simulink library "thc"  (R2021b)
settings: Solver=VariableStepAuto  StartTime=0.0  StopTime=10.0  RelTol=1e-3
undefined symbols (not defined in the file): ATHC_APTCQA_X_C, ATHC_APTCQB_X_C, ATHC_dAy_X_C, ATHC_Qeq_X_kmh, ATHC_VbaseC_X_C, ATHC_VbaseC_Y_W, ATHC_VbaseD_X_C, ATHC_VbaseH_X_C, FALSE, KTHC_ACMaxMinT_sec, KTHC_aDeice_K, KTHC_AGSDefLv_K, KTHC_AGSLv1_K, KTHC_AGSLv2_K, KTHC_AGSLv3_K, KTHC_AGSLv4_K, KTHC_AGSLv5_K, KTHC_AirIntUpdateT_sec, KTHC_APTCOneZoneMax_W, KTHC_APTCPeriod_cnt, KTHC_APTCPWMEN_flg, KTHC_APTCQMaxC_W, KTHC_APTCQminC_W, KTHC_APTCQminD_W, KTHC_APTCQminRe1_W, KTHC_APTCQminRe_W, KTHC_APTCQoffT_cnt, KTHC_APTCQonT_cnt, KTHC_APTCRiLeMaxDff_W, KTHC_APTCRiLeMinDff_W, KTHC_BatCoolT_cnt, KTHC_BatInTempDef_C, KTHC_bDeice_K, KTHC_CompMaxDeice_rpm, KTHC_CompMinDeice_rpm, KTHC_CompSotxvOp_K, KTHC_CompSotxvOpLow_rpm, KTHC_CompSpdmax_rpm, KTHC_CompSpdmaxBC1_rpm, KTHC_CompSpdmaxBC_rpm, KTHC_CompSpdmid1_rpm, KTHC_CompSpdmid2_rpm, KTHC_CompSpdmid3_rpm, KTHC_CompSpdmid_rpm, KTHC_CompSpdmin_rpm, KTHC_DAPTCQ1_W, KTHC_DAPTCQ2_W, KTHC_DAPTCQ3_W, KTHC_DcChSetTemp_C, KTHC_DehumidityEN_flg, KTHC_DeiceCycTime_K, KTHC_DriveLevelWPTCBAH1_W, KTHC_DriveLevelWPTCBAH2_W, KTHC_DriveLevelWPTCBAH3_W, KTHC_DriveLevelWPTCBAH4_W, KTHC_DriverSeatPos_flg, KTHC_DriveT1MinBAH_C, KTHC_DriveT2MaxBAH_C, KTHC_DriveT2MinBAH_C, KTHC_DriveT3MaxBAH_C ... (+379)
libraries: simulink x489
(part 13 of 17)

== system thc/THC/ThermalControl/THCM_Conctrl/EXV2Ctrl ==
  EXV2SHSetpoint : Inport
  PT_ Low_T2 : Inport  Port=2
  PT_ Low_P2 : Inport  Port=3
  EXV2PIDMode : Inport  Port=4
  EXVOpen : Inport  Port=5
  ErrEXV2FroceOFF : Inport  Port=6
  Compare To Constant : simulink/Logic and Bit Operations/Compare To Constant  relop=>  const=0  OutDataTypeStr=boolean
  Compare To Constant1 : simulink/Logic and Bit Operations/Compare To Constant  relop===  const=2  OutDataTypeStr=boolean
  Constant : Constant  Value=0.1
  Constant1 : Constant  Value=538
  Constant10 : Constant  Value=KTHC_EXVBlancePulse_K
  Constant11 : Constant  Value=ZERO_INT
  Constant12 : Constant  Value=KTHC_RefrigerantType_enum
  Constant2 : Constant  Value=38
  Constant3 : Constant  Value=0
  Constant4 : Constant  Value=0
  Constant5 : Constant  Value=KTHC_KpEXV2SH_K
  Constant6 : Constant  Value=KTHC_KiEXV2SH_K
  Constant7 : Constant  Value=0
  Constant8 : Constant  Value=KTHC_KpEXV2SHD_K
  Constant9 : Constant  Value=KTHC_KiEXV2SHD_K
  EXV2PIControl : Subsystem
  Gain : Gain  Gain=1/1000
  Multiport Switch : MultiPortSwitch  DataPortOrder=Zero-based contiguous  zeroidx=on
  Multiport Switch1 : MultiPortSwitch  DataPortOrder=Zero-based contiguous  zeroidx=on
  Multiport Switch2 : MultiPortSwitch  DataPortOrder=Zero-based contiguous  zeroidx=on
  Product : Product
  R1234yf : Lookup_n-D  NumberOfTableDimensions=1  BreakpointsForDimension1=[0.03742 0.06237 0.09906 0.11778 0.15092 0.1909 0.2386 0.29495 0.36092 0.43753 0.52583 0.6269 0.74189 0.87197 1.0184 1.3023]  Table=[-50 -40 -30 -26 -20 -14 -8 -2 4 10 16 22 28 34 40 50]  InternalRulePriority=Speed  RndMeth=Simplest  InputSameDT=on
  R134a : Lookup_n-D  NumberOfTableDimensions=1  BreakpointsForDimension1=[0.02945 0.05121 0.08438 0.10167 0.13273 0.17082 0.21693 0.27217 0.33766 0.41461 0.50425 0.60789 0.72688 0.86263 1.0166 1.31790]  Table=[-50 -40 -30 -26 -20 -14 -8 -2 4 10 16 22 28 34 40 50]  InternalRulePriority=Speed  RndMeth=Simplest  InputSameDT=on
  Saturation3 : Saturate  UpperLimit=1  LowerLimit=0
  Sum10 : Sum  Inputs=|++
  Sum7 : Sum  Inputs=|-+
  Sum8 : Sum  Inputs=|+-
  Sum9 : Sum  Inputs=|-+
  Switch : Switch  Criteria=u2 > Threshold
  Switch1 : Switch  Criteria=u2 > Threshold
  Switch2 : Switch  Criteria=u2 > Threshold
  Unit Delay1 : UnitDelay  SampleTime=-1  HasFrameUpgradeWarning=on
  EXV2 : Outport
  Tsat_low2 : Outport  Port=2
  VTHC_EXV2P_K : Outport  Port=3
  VTHC_EXV2I_K : Outport  Port=4
  VTHC_EXV2U_K : Outport  Port=5
  VTHC_EXV2e_K : Outport  Port=6
  wires:
  EXV2PIControl/3(VTHC_EXV2U_K) -> VTHC_EXV2U_K/1, Sum9/1  "U"
  Constant/1 -> Sum9/2
  Constant1/1 -> Product/2
  Sum9/1 -> Saturation3/1  "0.1-U"
  Gain/1 -> R1234yf/1, R134a/1
  Saturation3/1 -> Product/1  "EXV2%"
  Constant2/1 -> Sum10/1
  Sum7/1 -> Sum8/2  "SH"
  PT_ Low_T2/1 -> Sum7/2  "Tlow2"
  Sum10/1 -> Switch/1  "EXV2_Pulse"
  EXV2PIDMode/1 -> Switch1/3
  PT_ Low_P2/1 -> Gain/1
  EXV2SHSetpoint/1 -> Sum8/1
  Switch2/1 -> Tsat_low2/1, Sum7/1  "Tsat_low2"
  Sum8/1 -> VTHC_EXV2e_K/1, EXV2PIControl/1(x)  "e"
  Product/1 -> Sum10/2
  EXV2PIControl/1(VTHC_EXV2P_K) -> VTHC_EXV2P_K/1
  EXV2PIControl/2(VTHC_EXV2I_K) -> VTHC_EXV2I_K/1
  [EXV2PIDMode] -> EXV2PIControl/2(Reset)
  [EXV2PIDMode] -> Multiport Switch/1
  Constant4/1 -> Multiport Switch/2
  Constant7/1 -> Multiport Switch1/2
  [EXV2PIDMode] -> Multiport Switch1/1
  Multiport Switch/1 -> [KpEXV2]
  Constant5/1 -> Multiport Switch/3
  Constant8/1 -> Multiport Switch/4
  [KpEXV2] -> EXV2PIControl/3(VTHC_KpEXV2_K)
  Multiport Switch1/1 -> [KiEXV2]
  Constant6/1 -> Multiport Switch1/3
  Constant9/1 -> Multiport Switch1/4
  [KiEXV2] -> EXV2PIControl/4(VTHC_KiEXV2_K)
  [EXV2PIDMode] -> Compare To Constant/1
  Compare To Constant/1 -> Switch/2
  Constant3/1 -> Switch/3
  Multiport Switch2/1 -> Unit Delay1/1, EXV2/1  "EXV2_Pulse"
  Unit Delay1/1 -> Multiport Switch2/3
  EXVOpen/1 -> Multiport Switch2/1
  Constant10/1 -> Multiport Switch2/4
  Switch/1 -> Multiport Switch2/2
  ErrEXV2FroceOFF/1 -> Switch1/2
  Constant11/1 -> Switch1/1
  Switch1/1 -> [EXV2PIDMode]
  R1234yf/1 -> Switch2/1
  Constant12/1 -> Compare To Constant1/1
  Compare To Constant1/1 -> Switch2/2
  R134a/1 -> Switch2/3

== system thc/THC/ThermalControl/THCM_Conctrl/RadiatorFan ==
  FAN : Inport
  AGS_Err : Inport  Port=2
  AGS : Inport  Port=3
  Compare To Constant : simulink/Logic and Bit Operations/Compare To Constant  relop=>  const=1  OutDataTypeStr=boolean
  Constant : Constant  Value=KTHC_FANLv1_pct
  Constant1 : Constant  Value=KTHC_FANLv2_pct
  Constant2 : Constant  Value=KTHC_FANLv3_pct
  Constant3 : Constant  Value=KTHC_FANLv4_pct
  Constant4 : Constant  Value=KTHC_FANLv5_pct
  Constant5 : Constant  Value=0
  Constant6 : Constant  Value=KTHC_FANDefLv_pct
  Constant7 : Constant  Value=KTHC_ErrHandleEN_flg
  Logical Operator : Logic  Inputs=3  AllPortsSameDT=off  OutDataTypeStr=boolean
  Multiport Switch : MultiPortSwitch  Inputs=6  DiagnosticForDefault=None
  Switch : Switch  Criteria=u2 > Threshold
  CoolgFanActDuty : Outport
  wires:
  FAN/1 -> Multiport Switch/1
  Constant/1 -> Multiport Switch/2
  Constant5/1 -> Multiport Switch/7
  Constant4/1 -> Multiport Switch/6
  Constant1/1 -> Multiport Switch/3
  Constant2/1 -> Multiport Switch/4
  Constant3/1 -> Multiport Switch/5
  Logical Operator/1 -> Switch/2
  Constant6/1 -> Switch/1
  AGS/1 -> Compare To Constant/1
  AGS_Err/1 -> Logical Operator/1
  Compare To Constant/1 -> Logical Operator/2
  Switch/1 -> CoolgFanActDuty/1
  Multiport Switch/1 -> Switch/3
  Constant7/1 -> Logical Operator/3

== system thc/THC/ThermalControl/THCM_Conctrl/SensorErrorHandle1 ==
  DataIn : Inport
  SensorError : Inport  Port=2
  PresetValue : Inport  Port=3
  Constant : Constant  Value=KTHC_ErrHandleEN_flg
  Logical Operator : Logic  AllPortsSameDT=off  OutDataTypeStr=boolean
  Switch : Switch  Criteria=u2 > Threshold
  DataOut : Outport
  wires:
  PresetValue/1 -> Switch/1
  DataIn/1 -> Switch/3
  Switch/1 -> DataOut/1
  Logical Operator/1 -> Switch/2
  SensorError/1 -> Logical Operator/1
  Constant/1 -> Logical Operator/2

== system thc/THC/ThermalControl/THCM_Conctrl/SensorErrorHandle10 ==
  DataIn : Inport
  SensorError : Inport  Port=2
  PresetValue : Inport  Port=3
  Constant : Constant  Value=KTHC_ErrHandleEN_flg
  Logical Operator : Logic  AllPortsSameDT=off  OutDataTypeStr=boolean
  Switch : Switch  Criteria=u2 > Threshold
  DataOut : Outport
  wires:
  Constant/1 -> Logical Operator/2
  SensorError/1 -> Logical Operator/1
  Logical Operator/1 -> Switch/2
  Switch/1 -> DataOut/1
  DataIn/1 -> Switch/3
  PresetValue/1 -> Switch/1

== system thc/THC/ThermalControl/THCM_Conctrl/SensorErrorHandle11 ==
  DataIn : Inport
  SensorError : Inport  Port=2
  PresetValue : Inport  Port=3
  Constant : Constant  Value=KTHC_ErrHandleEN_flg
  Logical Operator : Logic  AllPortsSameDT=off  OutDataTypeStr=boolean
  Switch : Switch  Criteria=u2 > Threshold
  DataOut : Outport
  wires:
  Constant/1 -> Logical Operator/2
  SensorError/1 -> Logical Operator/1
  Logical Operator/1 -> Switch/2
  Switch/1 -> DataOut/1
  DataIn/1 -> Switch/3
  PresetValue/1 -> Switch/1

== system thc/THC/ThermalControl/THCM_Conctrl/SensorErrorHandle12 ==
  DataIn : Inport
  SensorError : Inport  Port=2
  PresetValue : Inport  Port=3
  Constant : Constant  Value=KTHC_ErrHandleEN_flg
  Logical Operator : Logic  AllPortsSameDT=off  OutDataTypeStr=boolean
  Switch : Switch  Criteria=u2 > Threshold
  DataOut : Outport
  wires:
  Constant/1 -> Logical Operator/2
  SensorError/1 -> Logical Operator/1
  Logical Operator/1 -> Switch/2
  Switch/1 -> DataOut/1
  DataIn/1 -> Switch/3
  PresetValue/1 -> Switch/1

== system thc/THC/ThermalControl/THCM_Conctrl/SensorErrorHandle2 ==
  DataIn : Inport
  SensorError : Inport  Port=2
  PresetValue : Inport  Port=3
  Constant : Constant  Value=KTHC_ErrHandleEN_flg
  Logical Operator : Logic  AllPortsSameDT=off  OutDataTypeStr=boolean
  Switch : Switch  Criteria=u2 > Threshold
  DataOut : Outport
  wires:
  Constant/1 -> Logical Operator/2
  SensorError/1 -> Logical Operator/1
  Logical Operator/1 -> Switch/2
  Switch/1 -> DataOut/1
  DataIn/1 -> Switch/3
  PresetValue/1 -> Switch/1

== system thc/THC/ThermalControl/THCM_Conctrl/SensorErrorHandle3 ==
  DataIn : Inport
  SensorError : Inport  Port=2
  PresetValue : Inport  Port=3
  Constant : Constant  Value=KTHC_ErrHandleEN_flg
  Logical Operator : Logic  AllPortsSameDT=off  OutDataTypeStr=boolean
  Switch : Switch  Criteria=u2 > Threshold
  DataOut : Outport
  wires:
  PresetValue/1 -> Switch/1
  DataIn/1 -> Switch/3
  Switch/1 -> DataOut/1
  Logical Operator/1 -> Switch/2
  SensorError/1 -> Logical Operator/1
  Constant/1 -> Logical Operator/2

== system thc/THC/ThermalControl/THCM_Conctrl/SensorErrorHandle4 ==
  DataIn : Inport
  SensorError : Inport  Port=2
  PresetValue : Inport  Port=3
  Constant : Constant  Value=KTHC_TevaErrHandleEN_flg
  Logical Operator : Logic  AllPortsSameDT=off  OutDataTypeStr=boolean
  Switch : Switch  Criteria=u2 > Threshold
  DataOut : Outport
  wires:
  PresetValue/1 -> Switch/1
  DataIn/1 -> Switch/3
  Switch/1 -> DataOut/1
  Logical Operator/1 -> Switch/2
  SensorError/1 -> Logical Operator/1
  Constant/1 -> Logical Operator/2

== system thc/THC/ThermalControl/THCM_Conctrl/SensorErrorHandle5 ==
  DataIn : Inport
  SensorError : Inport  Port=2
  PresetValue : Inport  Port=3
  Constant : Constant  Value=KTHC_TevaErrHandleEN_flg
  Logical Operator : Logic  AllPortsSameDT=off  OutDataTypeStr=boolean
  Switch : Switch  Criteria=u2 > Threshold
  DataOut : Outport
  wires:
  Constant/1 -> Logical Operator/2
  SensorError/1 -> Logical Operator/1
  Logical Operator/1 -> Switch/2
  Switch/1 -> DataOut/1
  DataIn/1 -> Switch/3
  PresetValue/1 -> Switch/1

== system thc/THC/ThermalControl/THCM_Conctrl/SensorErrorHandle6 ==
  DataIn : Inport
  SensorError : Inport  Port=2
  PresetValue : Inport  Port=3
  Constant : Constant  Value=KTHC_TevaErrHandleEN_flg
  Logical Operator : Logic  AllPortsSameDT=off  OutDataTypeStr=boolean
  Switch : Switch  Criteria=u2 > Threshold
  DataOut : Outport
  wires:
  PresetValue/1 -> Switch/1
  DataIn/1 -> Switch/3
  Switch/1 -> DataOut/1
  Logical Operator/1 -> Switch/2
  SensorError/1 -> Logical Operator/1
  Constant/1 -> Logical Operator/2

== system thc/THC/ThermalControl/THCM_Conctrl/SensorErrorHandle7 ==
  DataIn : Inport
  SensorError : Inport  Port=2
  PresetValue : Inport  Port=3
  Constant : Constant  Value=KTHC_TevaErrHandleEN_flg
  Logical Operator : Logic  AllPortsSameDT=off  OutDataTypeStr=boolean
  Switch : Switch  Criteria=u2 > Threshold
  DataOut : Outport
  wires:
  Constant/1 -> Logical Operator/2
  SensorError/1 -> Logical Operator/1
  Logical Operator/1 -> Switch/2
  Switch/1 -> DataOut/1
  DataIn/1 -> Switch/3
  PresetValue/1 -> Switch/1

== system thc/THC/ThermalControl/THCM_Conctrl/SensorErrorHandle8 ==
  DataIn : Inport
  SensorError : Inport  Port=2
  PresetValue : Inport  Port=3
  Constant : Constant  Value=KTHC_TevaErrHandleEN_flg
  Logical Operator : Logic  AllPortsSameDT=off  OutDataTypeStr=boolean
  Switch : Switch  Criteria=u2 > Threshold
  DataOut : Outport
  wires:
  PresetValue/1 -> Switch/1
  DataIn/1 -> Switch/3
  Switch/1 -> DataOut/1
  Logical Operator/1 -> Switch/2
  SensorError/1 -> Logical Operator/1
  Constant/1 -> Logical Operator/2

== system thc/THC/ThermalControl/THCM_Conctrl/SensorErrorHandle9 ==
  DataIn : Inport
  SensorError : Inport  Port=2
  PresetValue : Inport  Port=3
  Constant : Constant  Value=KTHC_TevaErrHandleEN_flg
  Logical Operator : Logic  AllPortsSameDT=off  OutDataTypeStr=boolean
  Switch : Switch  Criteria=u2 > Threshold
  DataOut : Outport
  wires:
  Constant/1 -> Logical Operator/2
  SensorError/1 -> Logical Operator/1
  Logical Operator/1 -> Switch/2
  Switch/1 -> DataOut/1
  DataIn/1 -> Switch/3
  PresetValue/1 -> Switch/1

== system thc/THC/ThermalControl/THCM_Conctrl/Subsystem ==
  CompSpd : Inport
  CabinMode : Inport  Port=2
  CompFB : Inport  Port=3
  Chart : Stateflow chart  TreatAsAtomicUnit=on
      settings: PortSchema="{\"entries\":[{\"content\":{\"sides\":[{\"content\":{\"connectorIds\":[\"In7\",\"In1\",\"In2\",\"In3\",\"In4\",\"In5\",\"In6\",\"In8\",\"In9\",\"In10\",\"In11\"]},\"type\":\"ConnectorPlacement.EquallySpacedRectSide\",\"uuid\":\"1db6d48d-2993-4fd1-a317-039acf53791d\"},{\"content\":{\"connectorIds\":[\"Out1\",\"Out2\",\"Out3\"],\"side\":\"RIGHT\"},\"type\":\"ConnectorPlacement.EquallySpacedRectSide\",\"uuid\":\"3b07bc2c-8788-4d9a-bac7-12ac97bb3dfe\"},{\"content\":{\"connectorIds\":[],\"side\":\"TOP\"},\"type\":\"ConnectorPlacement.EquallySpacedRectSide\",\"uuid\":\"678ef0de-745c-42f5-bb8c-af17f8a0632e\"}]},\"type\":\"ConnectorPlacement.EquallySpacedConnector\",\"uuid\":\"729d42ab-7bc1-4f80-88b9-90079b8c4930\"}],\"packageUris\":[\"http://schema.mathworks.com/mf0/Connector/R2020b\"],\"version\":\"1.0\"}"
  Compare To Constant : simulink/Logic and Bit Operations/Compare To Constant  relop=>=  const=2  OutDataTypeStr=boolean
  Compare To Constant1 : simulink/Logic and Bit Operations/Compare To Constant  relop=>  const=3  OutDataTypeStr=boolean
  Compare To Constant10 : simulink/Logic and Bit Operations/Compare To Constant  relop=<  const=10  OutDataTypeStr=boolean
  Compare To Constant11 : simulink/Logic and Bit Operations/Compare To Constant  relop===  const=9  OutDataTypeStr=boolean
  Compare To Constant12 : simulink/Logic and Bit Operations/Compare To Constant  relop===  const=1  OutDataTypeStr=boolean
  Compare To Constant13 : simulink/Logic and Bit Operations/Compare To Constant  relop===  const=5  OutDataTypeStr=boolean
  Compare To Constant2 : simulink/Logic and Bit Operations/Compare To Constant  relop=>=  const=1  OutDataTypeStr=boolean
  Compare To Constant3 : simulink/Logic and Bit Operations/Compare To Constant  relop=<=  const=3  OutDataTypeStr=boolean
  Compare To Constant4 : simulink/Logic and Bit Operations/Compare To Constant  relop===  const=8  OutDataTypeStr=boolean
  Compare To Constant5 : simulink/Logic and Bit Operations/Compare To Constant  relop===  const=6  OutDataTypeStr=boolean
  Compare To Constant6 : simulink/Logic and Bit Operations/Compare To Constant  relop===  const=7  OutDataTypeStr=boolean
  Compare To Constant7 : simulink/Logic and Bit Operations/Compare To Constant  relop===  const=4  OutDataTypeStr=boolean
  Compare To Constant8 : simulink/Logic and Bit Operations/Compare To Constant  relop=~=  const=7  OutDataTypeStr=boolean
  Compare To Constant9 : simulink/Logic and Bit Operations/Compare To Constant  relop=>=  const=10  OutDataTypeStr=boolean
  Constant3 : Constant  Value=0
  Constant4 : Constant  Value=KTHC_PBlaceTime1_K
  Constant5 : Constant  Value=KTHC_PBlaceTime2_K
  Constant6 : Constant  Value=KTHC_PBlaceTime3_K
  Constant7 : Constant  Value=KTHC_PBlaceTime4_K
  Logical Operator : Logic  AllPortsSameDT=off  OutDataTypeStr=boolean
  Logical Operator1 : Logic  Operator=OR  Inputs=4  AllPortsSameDT=off  OutDataTypeStr=boolean
  Logical Operator2 : Logic  Operator=OR  Inputs=4  AllPortsSameDT=off  OutDataTypeStr=boolean
  Logical Operator3 : Logic  Operator=OR  AllPortsSameDT=off  OutDataTypeStr=boolean
  Logical Operator4 : Logic  Inputs=3  AllPortsSameDT=off  OutDataTypeStr=boolean
  Logical Operator7 : Logic  Operator=NOT  AllPortsSameDT=off  OutDataTypeStr=boolean
  Logical Operator8 : Logic  AllPortsSameDT=off  OutDataTypeStr=boolean
  NOT : Logic  Operator=NOT  IconShape=distinctive  AllPortsSameDT=off  OutDataTypeStr=boolean
  NOT1 : Logic  Operator=NOT  IconShape=distinctive  AllPortsSameDT=off  OutDataTypeStr=boolean
  NOT2 : Logic  Operator=NOT  IconShape=distinctive  AllPortsSameDT=off  OutDataTypeStr=boolean
  Switch{,2,4,6} (4 alike) : Switch  Criteria=u2 > Threshold
  Unit Delay{,1..5} (6 alike) : UnitDelay  SampleTime=-1  HasFrameUpgradeWarning=on
  FD_Comp_Cmd : Outport
  FD_SOV1_Cmd : Outport  Port=2
  FD_SOV2_Cmd : Outport  Port=3
  FD_SOV3_Cmd : Outport  Port=4
  EXVOpen : Outport  Port=5
  wires:
  Logical Operator1/1 -> Unit Delay/1, [SOV1C], Chart/1(SOV1C)
  Unit Delay/1 -> Chart/2(SOV1CBuf)
  Unit Delay1/1 -> Chart/4(SOV2CBuf)
  Logical Operator3/1 -> Unit Delay1/1, [SOV2C], Chart/3(SOV2C)
  Logical Operator2/1 -> [SOV3C], Chart/5(SOV3C), Unit Delay2/1
  Unit Delay2/1 -> Chart/6(SOV3CBuf)
  Unit Delay3/1 -> Switch/1
  Switch/1 -> Unit Delay3/1, NOT/1
  Chart/2(Keep) -> [Keep]
  [SOV1C] -> Switch/3
  [Keep] -> Switch/2
  [Keep] -> Switch2/2
  [SOV2C] -> Switch2/3
  Switch2/1 -> Unit Delay4/1, NOT1/1
  Unit Delay4/1 -> Switch2/1
  Unit Delay5/1 -> Switch4/1
  Switch4/1 -> Unit Delay5/1, NOT2/1
  [SOV3C] -> Switch4/3
  [Keep] -> Switch4/2
  NOT/1 -> FD_SOV1_Cmd/1  "FD_SOV1_Cmd"
  NOT1/1 -> FD_SOV2_Cmd/1  "FD_SOV2_Cmd"
  NOT2/1 -> FD_SOV3_Cmd/1  "FD_SOV3_Cmd"
  Logical Operator7/1 -> Logical Operator8/2
  CompSpd/1 -> Switch6/1
  Switch6/1 -> FD_Comp_Cmd/1  "FD_Comp_Cmd"
  Constant3/1 -> Switch6/3
  Logical Operator8/1 -> Switch6/2
  Chart/1(FCompOFF) -> Logical Operator7/1
  Compare To Constant12/1 -> Logical Operator3/1
  Compare To Constant3/1 -> Logical Operator/2
  Compare To Constant2/1 -> Logical Operator/1
  Compare To Constant1/1 -> Logical Operator4/1
  CompFB/1 -> Chart/7(Comp)
  Compare To Constant/1 -> Logical Operator8/1
  Logical Operator/1 -> Logical Operator1/1
  Compare To Constant5/1 -> Logical Operator1/2
  Compare To Constant6/1 -> Logical Operator1/3
  CabinMode/1 -> Compare To Constant5/1, Compare To Constant9/1, Compare To Constant11/1, Compare To Constant7/1, Compare To Constant13/1, Compare To Constant4/1, Compare To Constant10/1, Compare To Constant8/1, Compare To Constant1/1, Compare To Constant12/1, Compare To Constant6/1, Compare To Constant/1, Compare To Constant2/1, Compare To Constant3/1
  Compare To Constant7/1 -> Logical Operator2/3
  Logical Operator4/1 -> Logical Operator3/2
  Compare To Constant8/1 -> Logical Operator4/2
  Compare To Constant9/1 -> Logical Operator1/4
  Compare To Constant10/1 -> Logical Operator4/3
  Compare To Constant13/1 -> Logical Operator2/4
  Constant4/1 -> Chart/8(KTHC_PBlaceTime1_K)
  Constant5/1 -> Chart/9(KTHC_PBlaceTime2_K)
  Constant6/1 -> Chart/10(KTHC_PBlaceTime3_K)
  Chart/3(EXVOpen) -> EXVOpen/1
  Constant7/1 -> Chart/11(KTHC_PBlaceTime4_K)
  Compare To Constant11/1 -> Logical Operator2/2
  Compare To Constant4/1 -> Logical Operator2/1

== system thc/THC/ThermalControl/THCM_Conctrl/Subsystem1 ==
  T_Face_L : Inport
  T_Face_R : Inport  Port=2
  T_Foot_L : Inport  Port=3
  T_Foot_R : Inport  Port=4
  T_Face_Rr : Inport  Port=5
  T_Foot_Rr : Inport  Port=6
  T_Face_L_Err : Inport  Port=7
  T_Face_R_Err : Inport  Port=8
  T_Foot_L_Err : Inport  Port=9
  T_Foot_R_Err : Inport  Port=10
  T_Face_Rr_Err : Inport  Port=11
  T_Foot_Rr_Err : Inport  Port=12
  CabinMode : Inport  Port=13
  Tincar : Inport  Port=14
  Tincar_Err : Inport  Port=15
  ACSubMode : Inport  Port=16
  Add : Sum  Inputs=++++++
  Add1 : Sum  Inputs=++++++
  Add2 : Sum
  Compare To Constant : simulink/Logic and Bit Operations/Compare To Constant  relop=<  const=4  OutDataTypeStr=boolean
  Compare To Constant1 : simulink/Logic and Bit Operations/Compare To Constant  relop=<  const=8  OutDataTypeStr=boolean
  Compare To Constant2 : simulink/Logic and Bit Operations/Compare To Constant  relop=~=  const=0  OutDataTypeStr=boolean
  Compare To Constant3 : simulink/Logic and Bit Operations/Compare To Constant  relop===  const=6  OutDataTypeStr=boolean
  Compare To Constant4 : simulink/Logic and Bit Operations/Compare To Constant  relop===  const=2  OutDataTypeStr=boolean
  Constant1 : Constant  Value=KTHC_TdiffC_C
  Constant{134..139} (6 alike) : Constant  Value=0
  Constant2 : Constant  Value=KTHC_TdiffD_C
  Constant3 : Constant  Value=KTHC_TdiffH_C
  Constant4 : Constant  Value=KTHC_TductDef_C
  Data Type Conversion{,1..7} (8 alike) : DataTypeConversion
  Divide : Product  Inputs=*/
  Logical Operator : Logic  Operator=OR  AllPortsSameDT=off  OutDataTypeStr=boolean
  Logical Operator1 : Logic  AllPortsSameDT=off  OutDataTypeStr=boolean
  NOT{,1..5} (6 alike) : Logic  Operator=NOT  IconShape=distinctive  AllPortsSameDT=off  OutDataTypeStr=boolean
  SensorErrorHandle1 : Subsystem
  SensorErrorHandle2 : Subsystem
  SensorErrorHandle3 : Subsystem
  SensorErrorHandle4 : Subsystem
  SensorErrorHandle5 : Subsystem
  SensorErrorHandle9 : Subsystem
  Switch{,1..3} (4 alike) : Switch  Criteria=u2 > Threshold
  Unit Delay : UnitDelay  SampleTime=-1  HasFrameUpgradeWarning=on
  Unit Delay1 : UnitDelay  SampleTime=-1  HasFrameUpgradeWarning=on
  TincarFix : Outport
  wires:
  T_Foot_L_Err/1 -> [T_Foot_L_Err]
  T_Face_R/1 -> SensorErrorHandle4/1(DataIn)
  T_Foot_R_Err/1 -> [T_Foot_R_Err]
  T_Foot_R/1 -> SensorErrorHandle2/1(DataIn)
  T_Foot_L/1 -> SensorErrorHandle3/1(DataIn)
  T_Face_R_Err/1 -> [T_Face_R_Err]
  T_Face_Rr/1 -> SensorErrorHandle1/1(DataIn)
  T_Foot_Rr/1 -> SensorErrorHandle9/1(DataIn)
  T_Foot_Rr_Err/1 -> [T_Foot_Rr_Err]
  T_Face_Rr_Err/1 -> [T_Face_Rr_Err]
  T_Face_L_Err/1 -> [T_Face_L_Err]
  [T_Face_R_Err] -> SensorErrorHandle4/2(SensorError)
  Constant135/1 -> SensorErrorHandle4/3(PresetValue)
  [T_Foot_L_Err] -> SensorErrorHandle3/2(SensorError)
  Constant136/1 -> SensorErrorHandle3/3(PresetValue)
  [T_Foot_R_Err] -> SensorErrorHandle2/2(SensorError)
  Constant137/1 -> SensorErrorHandle2/3(PresetValue)
  [T_Face_L_Err] -> SensorErrorHandle5/2(SensorError)
  Constant134/1 -> SensorErrorHandle5/3(PresetValue)
  T_Face_L/1 -> SensorErrorHandle5/1(DataIn)
  [T_Face_Rr_Err] -> SensorErrorHandle1/2(SensorError)
  Constant138/1 -> SensorErrorHandle1/3(PresetValue)
  [T_Foot_Rr_Err] -> SensorErrorHandle9/2(SensorError)
  Constant139/1 -> SensorErrorHandle9/3(PresetValue)
  SensorErrorHandle5/1(DataOut) -> Add/1
  SensorErrorHandle9/1(DataOut) -> Add/6
  SensorErrorHandle2/1(DataOut) -> Add/4
  SensorErrorHandle1/1(DataOut) -> Add/5
  SensorErrorHandle3/1(DataOut) -> Add/3
  SensorErrorHandle4/1(DataOut) -> Add/2
  Data Type Conversion/1 -> Add1/1
  NOT/1 -> Data Type Conversion/1
  [T_Face_L_Err] -> NOT/1
  [T_Face_R_Err] -> NOT1/1
  NOT1/1 -> Data Type Conversion1/1
  Data Type Conversion1/1 -> Add1/2
  NOT2/1 -> Data Type Conversion2/1
  [T_Foot_L_Err] -> NOT2/1
  Data Type Conversion2/1 -> Add1/3
  Data Type Conversion3/1 -> Add1/4
  [T_Foot_R_Err] -> NOT3/1
  NOT3/1 -> Data Type Conversion3/1
  NOT4/1 -> Data Type Conversion4/1
  [T_Face_Rr_Err] -> NOT4/1
  Data Type Conversion4/1 -> Add1/5
  Data Type Conversion5/1 -> Add1/6
  [T_Foot_Rr_Err] -> NOT5/1
  NOT5/1 -> Data Type Conversion5/1
  Add/1 -> Divide/1
  Add1/1 -> Compare To Constant2/1, Divide/2
  CabinMode/1 -> Unit Delay/1
  Unit Delay/1 -> Compare To Constant3/1, Compare To Constant1/1, Compare To Constant/1
  Switch1/1 -> Switch/3
  Compare To Constant1/1 -> Switch1/2
  Constant1/1 -> Switch/1
  Constant2/1 -> Switch1/1
  Constant3/1 -> Switch1/3
  Compare To Constant2/1 -> Switch2/2
  Divide/1 -> Data Type Conversion7/1
  Constant4/1 -> Switch2/3
  Switch2/1 -> Add2/1
  Switch/1 -> Add2/2
  Tincar_Err/1 -> Switch3/2
  Add2/1 -> Data Type Conversion6/1
  Tincar/1 -> Switch3/3
  Switch3/1 -> TincarFix/1
  Data Type Conversion6/1 -> Switch3/1
  Data Type Conversion7/1 -> Switch2/1
  Compare To Constant/1 -> Logical Operator/2
  Logical Operator/1 -> Switch/2
  ACSubMode/1 -> Unit Delay1/1
  Compare To Constant4/1 -> Logical Operator1/1
  Logical Operator1/1 -> Logical Operator/1
  Compare To Constant3/1 -> Logical Operator1/2
  Unit Delay1/1 -> Compare To Constant4/1

== system thc/THC/ThermalControl/THCM_Conctrl/Subsystem2 ==
  Motor_In_Temp : Inport
  Motor_In_Temp_Err : Inport  Port=2
  TBMax : Inport  Port=3
  Compare To Constant : simulink/Logic and Bit Operations/Compare To Constant  relop=>  const=20  OutDataTypeStr=boolean
  Constant1 : Constant  Value=KTHC_MotorInTempDefL_C
  Constant140 : Constant  Value=KTHC_MotorInTempDefH_C
  SensorErrorHandle9 : Subsystem
  Switch : Switch  Criteria=u2 > Threshold
  Motor_In_TempFix : Outport
  wires:
  TBMax/1 -> Compare To Constant/1
  Compare To Constant/1 -> Switch/2
  Constant140/1 -> Switch/1
  Constant1/1 -> Switch/3
  Motor_In_Temp/1 -> SensorErrorHandle9/1(DataIn)
  Motor_In_Temp_Err/1 -> SensorErrorHandle9/2(SensorError)
  Switch/1 -> SensorErrorHandle9/3(PresetValue)
  SensorErrorHandle9/1(DataOut) -> Motor_In_TempFix/1

== system thc/THC/ThermalControl/THCM_Conctrl/Subsystem3 ==
  note: 50
  FWVin : Inport
  TWVin : Inport  Port=2
  EWP1in : Inport  Port=3
  EWP2in : Inport  Port=4
  EWP3in : Inport  Port=5
  BalanceSW : Inport  Port=6
  "VINP_EWP1BlockError_enum " : Inport  Port=7
  VINP_EWP1OverCurrError_enum : Inport  Port=8
  VINP_EWP2BlockError_enum : Inport  Port=9
  VINP_EWP2OverCurrError_enum : Inport  Port=10
  VINP_EWP3BlockError_enum : Inport  Port=11
  VINP_EWP3OverCurrError_enum : Inport  Port=12
  Chart : Stateflow chart  TreatAsAtomicUnit=on
  Constant : Constant  Value=240
  Constant1 : Constant  Value=KTHC_ValueSWT_cnt
  Constant2 : Constant
  Constant3 : Constant  Value=0
  Constant4 : Constant  Value=0
  Constant5 : Constant  Value=0
  Constant9 : Constant  Value=KTHC_EWPStopT_cnt
  Data Type Conversion{,1..2,4..7} (7 alike) : DataTypeConversion  OutDataTypeStr=uint8
  Data Type Conversion3 : DataTypeConversion  OutDataTypeStr=boolean
  Detect Change : simulink/Logic and Bit Operations/Detect Change  vinit=0  OutDataTypeStr=boolean
  Detect Change1 : simulink/Logic and Bit Operations/Detect Change  vinit=0  OutDataTypeStr=boolean
  Logical Operator{,2,5..10} (8 alike) : Logic  AllPortsSameDT=off  OutDataTypeStr=boolean
  Logical Operator1 : Logic  Operator=OR  AllPortsSameDT=off  OutDataTypeStr=boolean
  Logical Operator11 : Logic  Operator=OR  Inputs=3  AllPortsSameDT=off  OutDataTypeStr=boolean
  Logical Operator3 : Logic  Operator=NOT  AllPortsSameDT=off  OutDataTypeStr=boolean
  Logical Operator4 : Logic  Operator=OR  AllPortsSameDT=off  OutDataTypeStr=boolean
  Max : MinMax  Function=max  Inputs=3
  Subsystem1 : Subsystem
  Subsystem2 : Subsystem
  Subsystem3 : Subsystem
  Switch{,1..12} (13 alike) : Switch  Criteria=u2 > Threshold
  Unit Delay{,1..7} (8 alike) : UnitDelay  SampleTime=-1  HasFrameUpgradeWarning=on
  FWV : Outport
  TWV : Outport  Port=2
  EWP1 : Outport  Port=3
  EWP2 : Outport  Port=4
  EWP3 : Outport  Port=5
  VTHC_EWPBUflag1_flg : Outport  Port=6
  VTHC_EWPBUflag2_flg : Outport  Port=7
  VTHC_EWPBUflag3_flg : Outport  Port=8
  VTHC_THSysErrlampReq_flg : Outport  Port=9
  wires:
  [FWVForceON] -> VTHC_THSysErrlampReq_flg/1  "VTHC_THSysErrlampReq_flg"
  [EWP3] -> Switch12/3
  Constant5/1 -> Data Type Conversion7/1
  Data Type Conversion7/1 -> Switch12/1
  [EWP3pause] -> Switch12/2
  Switch12/1 -> EWP3/1
  Switch11/1 -> EWP2/1
  [EWP2] -> Switch11/3
  Data Type Conversion6/1 -> Switch11/1
  Constant4/1 -> Data Type Conversion6/1
  [EWP2pause] -> Switch11/2
  Data Type Conversion5/1 -> Switch10/1
  Constant3/1 -> Data Type Conversion5/1
  [EWP1] -> Switch10/3
  [EWP1pause] -> Switch10/2
  Switch10/1 -> EWP1/1
  Subsystem2/3(EWPBUflag) -> VTHC_EWPBUflag3_flg/1
  Subsystem1/3(EWPBUflag) -> VTHC_EWPBUflag2_flg/1
  Subsystem2/2(EWPpause) -> [EWP3pause]
  Subsystem1/2(EWPpause) -> [EWP2pause]
  Subsystem3/3(EWPBUflag) -> VTHC_EWPBUflag1_flg/1
  Subsystem3/2(EWPpause) -> [EWP1pause]
  Data Type Conversion4/1 -> Detect Change1/1
  Constant2/1 -> Data Type Conversion3/1
  Data Type Conversion3/1 -> Switch9/1
  [FWVForceON] -> Switch9/2
  Switch9/1 -> [FWVin]
  Constant/1 -> Data Type Conversion2/1
  Data Type Conversion2/1 -> Switch8/1
  [FWVForceON] -> Switch8/2
  Max/1 -> Switch8/3
  Logical Operator11/1 -> [FWVForceON]
  [EWP3error] -> Logical Operator11/3
  [EWP2error] -> Logical Operator11/2
  [EWP1error] -> Logical Operator11/1
  Subsystem2/1(EWPerror) -> [EWP3error]
  Subsystem1/1(EWPerror) -> [EWP2error]
  VINP_EWP3OverCurrError_enum/1 -> Subsystem2/2(VINP_EWPOverCurrError_enum)
  VINP_EWP3BlockError_enum/1 -> Subsystem2/1("VINP_EWPBlockError_enum ")
  VINP_EWP2OverCurrError_enum/1 -> Subsystem1/2(VINP_EWPOverCurrError_enum)
  VINP_EWP2BlockError_enum/1 -> Subsystem1/1("VINP_EWPBlockError_enum ")
  VINP_EWP1OverCurrError_enum/1 -> Subsystem3/2(VINP_EWPOverCurrError_enum)
  "VINP_EWP1BlockError_enum "/1 -> Subsystem3/1("VINP_EWPBlockError_enum ")
  Subsystem3/1(EWPerror) -> [EWP1error]
  [BalanceSW] -> Logical Operator10/1
  [EWPKeep] -> Logical Operator10/2
  Logical Operator10/1 -> Switch6/2
  [BalanceSW] -> Logical Operator9/1
  [EWPKeep] -> Logical Operator9/2
  Logical Operator9/1 -> Switch5/2
  [BalanceSW] -> Logical Operator8/1
  [EWPKeep] -> Logical Operator8/2
  Logical Operator8/1 -> Switch4/2
  [BalanceSW] -> Logical Operator7/1
  Logical Operator4/1 -> Logical Operator7/2
  [BalanceSW] -> Logical Operator6/1
  [FWVKeep] -> Logical Operator6/2
  Logical Operator6/1 -> Switch1/2
  [TWVKeep] -> Logical Operator5/2
  [BalanceSW] -> Logical Operator5/1
  Logical Operator5/1 -> Switch/2
  BalanceSW/1 -> [BalanceSW]
  Switch6/1 -> Unit Delay7/1, [EWP3]
  Unit Delay7/1 -> Switch6/1
  Switch7/1 -> Switch6/3
  Switch3/1 -> Switch5/3
  Unit Delay6/1 -> Switch5/1
  Switch5/1 -> Unit Delay6/1, [EWP2]
  Switch4/1 -> [EWP1], Unit Delay5/1
  Unit Delay5/1 -> Switch4/1
  Chart/3(EWPKeep) -> [EWPKeep]
  Data Type Conversion1/1 -> Chart/7(ValueSWT)
  Constant1/1 -> Data Type Conversion1/1
  EWP3in/1 -> [EWP3in]
  EWP2in/1 -> [EWP2in]
  EWP1in/1 -> [EWP1in]
  [AllStopReq] -> Chart/2(AllStopReq)
  [PartStopReq] -> Chart/1(PartStopReq)
  [FWV] -> Logical Operator4/2
  [FWVin] -> Logical Operator4/1
  [FWV] -> FWV/1
  [EWP1] -> Unit Delay2/1
  Switch/1 -> Unit Delay3/1, TWV/1
  Chart/1(TWVKeep) -> [TWVKeep]
  [EWP3] -> Unit Delay/1
  Detect Change/1 -> Logical Operator1/1
  Data Type Conversion/1 -> Chart/6(EWPStopT)
  Logical Operator3/1 -> Logical Operator2/2
  [FWVin] -> Logical Operator3/1
  Unit Delay/1 -> Chart/5(EWP3)
  Unit Delay2/1 -> Chart/3(EWP1)
  [TWVin] -> Data Type Conversion4/1
  [EWP2in] -> Switch3/3
  [TWVin] -> Switch/3
  Logical Operator/1 -> Logical Operator1/2
  Switch2/1 -> Switch4/3
  [EWP2] -> Unit Delay1/1
  Detect Change1/1 -> Logical Operator/2, Logical Operator2/1
  Logical Operator2/1 -> [PartStopReq]
  [EWPMax] -> Switch2/1
  [EWP3in] -> Max/3
  FWVin/1 -> Switch9/3
  Switch8/1 -> [EWPMax]
  [EWP1in] -> Switch2/3
  Unit Delay1/1 -> Chart/4(EWP2)
  Logical Operator7/1 -> Switch2/2, Switch3/2, Switch7/2
  Chart/2(FWVKeep) -> [FWVKeep]
  Logical Operator1/1 -> [AllStopReq]
  TWVin/1 -> [TWVin]
  Constant9/1 -> Data Type Conversion/1
  [EWP1in] -> Max/1
  Unit Delay3/1 -> Switch/1
  [EWPMax] -> Switch3/1
  [EWP3in] -> Switch7/3
  [EWPMax] -> Switch7/1
  [FWVin] -> Logical Operator/1, Detect Change/1
  Unit Delay4/1 -> Switch1/1
  Switch1/1 -> [FWV], Unit Delay4/1
  [FWVin] -> Switch1/3
  [EWP2in] -> Max/2

== system thc/THC/ThermalControl/THCM_Conctrl/Subsystem4 ==
  sigSetTempZon1St : Inport
  Tamb : Inport  Port=2
  Add1 : Sum
  Add2 : Sum  Inputs=+-
  Constant : Constant  Value=0.5
  Constant1 : Constant  Value=0.5
  Constant2 : Constant
  Constant3 : Constant  Value=0
  Data Type Conversion : DataTypeConversion  OutDataTypeStr=single
  Data Type Conversion1 : DataTypeConversion  OutDataTypeStr=single
  Data Type Conversion2 : DataTypeConversion  OutDataTypeStr=boolean
  Data Type Conversion3 : DataTypeConversion  OutDataTypeStr=boolean
  Relational Operator : RelationalOperator  Operator=<=  OutDataTypeStr=boolean  RndMeth=Simplest
  Relational Operator1 : RelationalOperator  Operator=>  OutDataTypeStr=boolean  RndMeth=Simplest
  Switch : Switch  Criteria=u2 > Threshold
  Switch1 : Switch  Criteria=u2 > Threshold
  Unit Delay : UnitDelay  SampleTime=-1  HasFrameUpgradeWarning=on
  HeatReq : Outport
  wires:
  sigSetTempZon1St/1 -> [sigSetTempZon1St]
  Switch/1 -> Unit Delay/1, HeatReq/1
  Unit Delay/1 -> Switch1/3
  Switch1/1 -> Switch/3
  Data Type Conversion3/1 -> Switch1/1
  Constant3/1 -> Data Type Conversion3/1
  Relational Operator1/1 -> Switch1/2
  Add1/1 -> Relational Operator1/2
  [Tamb] -> Relational Operator1/1
  Data Type Conversion2/1 -> Switch/1
  Constant2/1 -> Data Type Conversion2/1
  Relational Operator/1 -> Switch/2
  Add2/1 -> Relational Operator/2
  [Tamb] -> Relational Operator/1
  Tamb/1 -> [Tamb]
  [sigSetTempZon1St] -> Add2/1
  Constant1/1 -> Data Type Conversion1/1
  Data Type Conversion1/1 -> Add2/2
  Data Type Conversion/1 -> Add1/2
  Constant/1 -> Data Type Conversion/1
  [sigSetTempZon1St] -> Add1/1

== system thc/THC/ThermalControl/THCM_Conctrl/WPTC ==
  WPTC : Inport
  EWP3_Err : Inport  Port=2
  PresetValue : Inport  Port=3
  Constant : Constant  Value=KTHC_ErrHandleEN_flg
  Logical Operator : Logic  AllPortsSameDT=off  OutDataTypeStr=boolean
  Switch : Switch  Criteria=u2 > Threshold
  DataOut : Outport
  wires:
  Switch/1 -> DataOut/1
  WPTC/1 -> Switch/3
  PresetValue/1 -> Switch/1
  Constant/1 -> Logical Operator/2
  EWP3_Err/1 -> Logical Operator/1
  Logical Operator/1 -> Switch/2

== system thc/THC/ThermalControl/THCM_Conctrl/APTC/APTCPIControl ==
  x : Inport
  Reset : Inport  Port=2
  CtrlReset : Inport  Port=3
  VTHC_KpAPTC_K : Inport  Port=4
  VTHC_KiAPTC_K : Inport  Port=5
  Add : Sum
  Add1 : Sum
  Constant : Constant  Value=0
  Equal : RelationalOperator  Operator=~=  OutDataTypeStr=boolean  RndMeth=Simplest
  Logical Operator : Logic  Operator=OR  AllPortsSameDT=off  OutDataTypeStr=boolean
  Product : Product
  Product1 : Product
  Saturation : Saturate  UpperLimit=1  LowerLimit=0
  Switch : Switch  Criteria=u2 > Threshold
  Ts : Gain  Gain=0.1
  Unit Delay : UnitDelay  SampleTime=-1  HasFrameUpgradeWarning=on
  Unit Delay1 : UnitDelay  SampleTime=-1  HasFrameUpgradeWarning=on
  VTHC_APTCP_K : Outport
  VTHC_APTCI_K : Outport  Port=2
  VTHC_APTCU_K : Outport  Port=3
  wires:
  Unit Delay/1 -> Equal/2
  Equal/1 -> Logical Operator/1
  Constant/1 -> Switch/1
  Product/1 -> VTHC_APTCP_K/1, Add/1  "VTHC_APTCP_K"
  Add/1 -> VTHC_APTCU_K/1
  Switch/1 -> VTHC_APTCI_K/1, Add/2, Add1/2  "VTHC_APTCI_K"
  Unit Delay1/1 -> Saturation/1
  Reset/1 -> Unit Delay/1, Equal/1
  VTHC_KpAPTC_K/1 -> Product/1
  VTHC_KiAPTC_K/1 -> Product1/1
  Saturation/1 -> Switch/3
  x/1 -> Product/2, Product1/2
  Add1/1 -> Unit Delay1/1
  Product1/1 -> Ts/1
  Ts/1 -> Add1/1  "VTHC_APTCI_K"
  CtrlReset/1 -> Logical Operator/2
  Logical Operator/1 -> Switch/2

== system thc/THC/ThermalControl/THCM_Conctrl/APTC/APTCPWMControl ==
  Win : Inport
  Chart : Stateflow chart  TreatAsAtomicUnit=on
  Constant : Constant  Value=KTHC_APTCPeriod_cnt
  Constant1 : Constant  Value=KTHC_APTCQminC_W
  Constant43 : Constant  Value=KTHC_APTCPWMEN_flg
  Data Type Conversion : DataTypeConversion  OutDataTypeStr=uint16
  Data Type Conversion1 : DataTypeConversion  OutDataTypeStr=uint16
  Data Type Conversion2 : DataTypeConversion  OutDataTypeStr=uint16
  Out1 : Outport
  wires:
  Constant43/1 -> Chart/4(KTHC_APTCPWMEN_flg)
  Win/1 -> Data Type Conversion/1  "Win"
  Chart/1(Wout) -> Out1/1  "Wout"
  Data Type Conversion1/1 -> Chart/2(Tp)
  Data Type Conversion2/1 -> Chart/3(Wmin)
  Constant/1 -> Data Type Conversion1/1
  Constant1/1 -> Data Type Conversion2/1
  Data Type Conversion/1 -> Chart/1(Win)

== system thc/THC/ThermalControl/THCM_Conctrl/APTC/APTCPWMControl1 ==
  Win : Inport
  Chart : Stateflow chart  TreatAsAtomicUnit=on
  Constant : Constant  Value=KTHC_APTCPeriod_cnt
  Constant1 : Constant  Value=KTHC_APTCQminC_W
  Constant43 : Constant  Value=KTHC_APTCPWMEN_flg
  Data Type Conversion : DataTypeConversion  OutDataTypeStr=uint16
  Data Type Conversion1 : DataTypeConversion  OutDataTypeStr=uint16
  Data Type Conversion2 : DataTypeConversion  OutDataTypeStr=uint16
  Out1 : Outport
  wires:
  Data Type Conversion/1 -> Chart/1(Win)
  Constant1/1 -> Data Type Conversion2/1
  Constant/1 -> Data Type Conversion1/1
  Data Type Conversion2/1 -> Chart/3(Wmin)
  Data Type Conversion1/1 -> Chart/2(Tp)
  Chart/1(Wout) -> Out1/1  "Wout"
  Win/1 -> Data Type Conversion/1  "Win"
  Constant43/1 -> Chart/4(KTHC_APTCPWMEN_flg)

== system thc/THC/ThermalControl/THCM_Conctrl/APTC/APTCPWMControl2 ==
  Win : Inport
  Chart : Stateflow chart  TreatAsAtomicUnit=on
  Constant : Constant  Value=KTHC_APTCPeriod_cnt
  Constant1 : Constant  Value=KTHC_APTCQminC_W
  Constant43 : Constant  Value=KTHC_APTCPWMEN_flg
  Data Type Conversion : DataTypeConversion  OutDataTypeStr=uint16
  Data Type Conversion1 : DataTypeConversion  OutDataTypeStr=uint16
  Data Type Conversion2 : DataTypeConversion  OutDataTypeStr=uint16
  Out1 : Outport
  wires:
  Constant43/1 -> Chart/4(KTHC_APTCPWMEN_flg)
  Win/1 -> Data Type Conversion/1  "Win"
  Chart/1(Wout) -> Out1/1  "Wout"
  Data Type Conversion1/1 -> Chart/2(Tp)
  Data Type Conversion2/1 -> Chart/3(Wmin)
  Constant/1 -> Data Type Conversion1/1
  Constant1/1 -> Data Type Conversion2/1
  Data Type Conversion/1 -> Chart/1(Win)

== system thc/THC/ThermalControl/THCM_Conctrl/APTC/Subsystem ==
  VehSpeed : Inport
  sigSetTempZon1St : Inport  Port=2
  sigSetTempZon2St : Inport  Port=3
  APTCQ : Inport  Port=4
  APTCPID : Inport  Port=5
  1-D Lookup Table : Lookup_n-D  NumberOfTableDimensions=1  BreakpointsForDimension1=ATHC_Qeq_X_kmh  Table=MTHC_Qeq_Y_K  InternalRulePriority=Speed  RndMeth=Simplest  InputSameDT=on
  Abs : Abs
  Add : Sum  Inputs=+-
  Add1 : Sum
  Add2 : Sum
  Add3 : Sum  Inputs=+--
  Add4 : Sum  Inputs=-+
  Compare To Constant : simulink/Logic and Bit Operations/Compare To Constant  relop=>=  const=0  OutDataTypeStr=boolean
  Compare To Constant1 : simulink/Logic and Bit Operations/Compare To Constant  relop=<  const=0  OutDataTypeStr=boolean
  Compare To Constant2 : simulink/Logic and Bit Operations/Compare To Constant  relop=>=  const=0  OutDataTypeStr=boolean
  Compare To Constant4 : simulink/Logic and Bit Operations/Compare To Constant  relop=<  const=0  OutDataTypeStr=boolean
  Constant{,1..5} (6 alike) : Constant  Value=0
  Constant6 : Constant  Value=KTHC_DriverSeatPos_flg
  Constant7 : Constant  Value=KTHC_DriverSeatPos_flg
  Gain : Gain  Gain=-1
  Gain1 : Gain  Gain=2
  Gain2 : Gain  Gain=1/3
  Product : Product
  Relational Operator : RelationalOperator  Operator=>  OutDataTypeStr=boolean  RndMeth=Simplest
  Saturation : Saturate  UpperLimit=KTHC_APTCRiLeMaxDff_W  LowerLimit=KTHC_APTCRiLeMinDff_W
  Saturation1 : Saturate  UpperLimit=KTHC_APTCOneZoneMax_W  LowerLimit=0
  Saturation2 : Saturate  UpperLimit=KTHC_APTCOneZoneMax_W  LowerLimit=0
  Switch{,1..11} (12 alike) : Switch  Criteria=u2 > Threshold
  FD_FrLeAPTC_Cmd : Outport
  FD_FrRiAPTC_Cmd : Outport  Port=2
  FD_RrAPTC_Cmd : Outport  Port=3
  wires:
  [APTCFrRiQ] -> Switch8/1
  [APTCFrLeQ] -> Switch7/1
  Switch10/1 -> [APTCFrRiQ]
  Switch11/1 -> [APTCFrLeQ]
  [APTCZ2Q] -> Switch11/1
  [APTCZ1Q] -> Switch11/3
  Constant7/1 -> Switch11/2
  Constant6/1 -> Switch10/2
  [APTCZ2Q] -> Switch10/3
  [APTCZ1Q] -> Switch10/1
  Switch2/1 -> [APTCZ2Q]
  [VTHC_APTC1stQ_W] -> Switch4/1
  VehSpeed/1 -> 1-D Lookup Table/1
  [APTCQTemp] -> Add3/1
  [qeq] -> Product/1
  Constant/1 -> Switch1/3
  1-D Lookup Table/1 -> [qeq]
  Gain1/1 -> Add1/2
  Saturation2/1 -> Switch5/3
  [APTCFrRiQ] -> Add3/3
  [Q12] -> Add2/1, Compare To Constant2/1
  Switch6/1 -> Switch2/3
  Switch4/1 -> Switch/3
  Saturation/1 -> [Q12], Abs/1
  Gain2/1 -> Saturation1/1
  Switch/1 -> [APTCZ1Q]
  [VTHC_APTC1stQ_W] -> Add4/2
  Add4/1 -> Switch6/3
  Constant2/1 -> Switch5/1
  Compare To Constant4/1 -> Switch6/2
  Compare To Constant/1 -> Switch1/2
  [APTCFrLeQ] -> Add3/2
  [VTHC_APTCZone1full_flg] -> Switch/2
  sigSetTempZon2St/1 -> Add/2
  [Q12] -> Switch1/1, Compare To Constant/1
  Relational Operator/1 -> [VTHC_APTCZone1full_flg]
  Add3/1 -> Saturation2/1
  [VTHC_APTCZone1full_flg] -> Switch2/2
  [Q12] -> Gain/1, Compare To Constant1/1
  [DTZone] -> Product/2
  Add/1 -> [DTZone]
  Abs/1 -> Gain1/1, Relational Operator/1
  Switch3/1 -> Switch2/1
  Compare To Constant2/1 -> Switch4/2
  Switch1/1 -> Switch/1
  [VTHC_APTC1stQ_W] -> Switch6/1
  [Q12] -> Add4/1, Compare To Constant4/1
  Compare To Constant1/1 -> Switch3/2
  sigSetTempZon1St/1 -> Add/1
  [VTHC_APTCZone1full_flg] -> Switch5/2
  Gain/1 -> Switch3/1
  [VTHC_APTC1stQ_W] -> Add2/2
  Product/1 -> Saturation/1
  [APTCQTemp] -> Add1/1, Relational Operator/2
  Add1/1 -> Gain2/1
  Add2/1 -> Switch4/3
  Constant1/1 -> Switch3/3
  Saturation1/1 -> [VTHC_APTC1stQ_W]
  Switch7/1 -> FD_FrLeAPTC_Cmd/1
  APTCPID/1 -> [APTCPID]
  Constant3/1 -> Switch7/3
  Constant4/1 -> Switch8/3
  [APTCPID] -> Switch8/2
  Switch8/1 -> FD_FrRiAPTC_Cmd/1
  Switch5/1 -> Switch9/1
  [APTCPID] -> Switch9/2
  Constant5/1 -> Switch9/3
  Switch9/1 -> FD_RrAPTC_Cmd/1
  APTCQ/1 -> [APTCQTemp]
  [APTCPID] -> Switch7/2

== system thc/THC/ThermalControl/THCM_Conctrl/BlowerCtrl/BlowerPIControl ==
  x : Inport
  Reset : Inport  Port=2
  VTHC_BlowerKp_K : Inport  Port=3
  VTHC_BlowerKi_K : Inport  Port=4
  Add : Sum
  Add1 : Sum
  Constant : Constant  Value=0
  Equal : RelationalOperator  Operator=~=  OutDataTypeStr=boolean  RndMeth=Simplest
  Product : Product
  Product1 : Product
  Saturation : Saturate  UpperLimit=1  LowerLimit=0
  Switch : Switch  Criteria=u2 > Threshold
  Ts : Gain  Gain=0.1
  Unit Delay : UnitDelay  SampleTime=-1  HasFrameUpgradeWarning=on
  Unit Delay1 : UnitDelay  SampleTime=-1  HasFrameUpgradeWarning=on
  VTHC_BlowerP_K : Outport
  VTHC_BlowerI_K : Outport  Port=2
  VTHC_BlowerU_K : Outport  Port=3
  wires:
  Reset/1 -> Unit Delay/1, Equal/1
  Unit Delay/1 -> Equal/2
  Equal/1 -> Switch/2
  Constant/1 -> Switch/1
  x/1 -> Product/2, Product1/1
  Product/1 -> VTHC_BlowerP_K/1, Add/1  "VTHC_BlowerP_K"
  Add/1 -> VTHC_BlowerU_K/1
  Add1/1 -> Unit Delay1/1
  Product1/1 -> Ts/1
  Switch/1 -> Add1/2, VTHC_BlowerI_K/1, Add/2  "VTHC_BlowerI_K"
  VTHC_BlowerKp_K/1 -> Product/1
  VTHC_BlowerKi_K/1 -> Product1/2
  Ts/1 -> Add1/1
  Unit Delay1/1 -> Saturation/1
  Saturation/1 -> Switch/3

== system thc/THC/ThermalControl/THCM_Conctrl/BlowerCtrl/Enabled Subsystem1 ==
  Blowersolar : Inport
  Tamb : Inport  Port=2
  CabinMode : Inport  Port=3
  ACAuto : Inport  Port=4
  Vmanual : Inport  Port=5
  DfrstReq : Inport  Port=6
  ACSubMode : Inport  Port=7
  PwrSta : Inport  Port=8
  1-D Lookup Table : Lookup_n-D  NumberOfTableDimensions=1  BreakpointsForDimension1=ATHC_VbaseH_X_C  Table=MTHC_VbaseH_Y_K  InternalRulePriority=Speed  RndMeth=Simplest  InputSameDT=on
  1-D Lookup Table1 : Lookup_n-D  NumberOfTableDimensions=1  BreakpointsForDimension1=ATHC_VbaseD_X_C  Table=MTHC_VbaseD_Y_K  InternalRulePriority=Speed  RndMeth=Simplest  InputSameDT=on
  2-D Lookup Table1 : Lookup_n-D  BreakpointsForDimension1=ATHC_VbaseC_Y_W  BreakpointsForDimension2=ATHC_VbaseC_X_C  Table=MTHC_VbaseC_Z_K  InternalRulePriority=Speed  RndMeth=Simplest  InputSameDT=on
      settings: InputPortMap=u0,u1
  Chart2 : Stateflow chart  TreatAsAtomicUnit=on
      settings: PortSchema="{\"entries\":[{\"content\":{\"sides\":[{\"content\":{\"connectorIds\":[\"In1\",\"In2\",\"In3\",\"In4\",\"In5\",\"In6\",\"In7\",\"In8\",\"In9\",\"In10\",\"In11\",\"In12\",\"In14\",\"In13\"]},\"type\":\"ConnectorPlacement.EquallySpacedRectSide\",\"uuid\":\"7e8f7538-56f4-447a-9145-c20cc29664fa\"},{\"content\":{\"connectorIds\":[\"Out1\"],\"side\":\"RIGHT\"},\"type\":\"ConnectorPlacement.EquallySpacedRectSide\",\"uuid\":\"8e6754a2-1b4c-4aa6-81e0-e2cdf3e8c159\"},{\"content\":{\"connectorIds\":[],\"side\":\"TOP\"},\"type\":\"ConnectorPlacement.EquallySpacedRectSide\",\"uuid\":\"22019b22-c6fe-41ab-ac44-688f1d70e28d\"}]},\"type\":\"ConnectorPlacement.EquallySpacedConnector\",\"uuid\":\"3c722edc-0b93-4b6c-89cb-f70cbb5ccb6e\"}],\"packageUris\":[\"http://schema.mathworks.com/mf0/Connector/R2020b\"],\"version\":\"1.0\"}"
  Constant : Constant  Value=KTHC_VBlowerdfog_K
  Constant1 : Constant  Value=KTHC_VBlowerMin_K
  Constant2 : Constant  Value=KTHC_VBlowerMid_K
  Constant3 : Constant  Value=KTHC_VBlowerSetLow_K
  Constant4 : Constant  Value=KTHC_VBlowerDcCh_K
  VBase : Outport
  wires:
  Tamb/1 -> [Tamb]
  1-D Lookup Table/1 -> Chart2/7(VbaseH)  "VBaseH"
  Blowersolar/1 -> 2-D Lookup Table1/1  "Blowersolar"
  [Tamb] -> 2-D Lookup Table1/2  "Tamb"
  2-D Lookup Table1/1 -> Chart2/5(VbaseC)  "VbaseC"
  [Tamb] -> 1-D Lookup Table/1  "Tamb"
  Vmanual/1 -> Chart2/8(Vmanual)
  CabinMode/1 -> Chart2/3(CabinMode)  "CabinMode"
  ACAuto/1 -> Chart2/1(ACAuto)
  Chart2/1(Voffset) -> VBase/1
  DfrstReq/1 -> Chart2/4(DfrstReq)
  ACSubMode/1 -> Chart2/2(ACSubMode)
  [Tamb] -> 1-D Lookup Table1/1  "Tamb"
  1-D Lookup Table1/1 -> Chart2/6(VbaseD)  "VBaseD"
  PwrSta/1 -> Chart2/9(PwrSta)
  Constant/1 -> Chart2/10(KTHC_VBlowerdfog_K)
  Constant1/1 -> Chart2/11(KTHC_VBlowerMin_K)
  Constant2/1 -> Chart2/12(KTHC_VBlowerMid_K)
  Constant3/1 -> Chart2/14(KTHC_VBlowerSetLow_K)
  Constant4/1 -> Chart2/13(KTHC_VBlowerDcCh_K)

== system thc/THC/ThermalControl/THCM_Conctrl/CompCtrl/CompPIControl ==
  x : Inport
  Reset : Inport  Port=2
  VTHC_CompKp_K : Inport  Port=3
  VTHC_CompKi_K : Inport  Port=4
  Add : Sum
  Add1 : Sum
  Compare To Constant : simulink/Logic and Bit Operations/Compare To Constant  relop=>  const=0  OutDataTypeStr=boolean
  Constant : Constant  Value=0
  Equal : RelationalOperator  Operator=~=  OutDataTypeStr=boolean  RndMeth=Simplest
  Logical Operator : Logic  AllPortsSameDT=off  OutDataTypeStr=boolean
  Product : Product
  Product1 : Product
  Switch : Switch  Criteria=u2 > Threshold
  Ts : Gain  Gain=0.1
  Unit Delay : UnitDelay  SampleTime=-1  HasFrameUpgradeWarning=on
  Unit Delay1 : UnitDelay  SampleTime=-1  HasFrameUpgradeWarning=on
  VTHC_CompP_K : Outport
  VTHC_CompI_K : Outport  Port=2
  VTHC_CompU_K : Outport  Port=3
  wires:
  Reset/1 -> Compare To Constant/1, Unit Delay/1, Equal/1
  Unit Delay/1 -> Equal/2
  Equal/1 -> Logical Operator/1
  Logical Operator/1 -> Switch/2
  Constant/1 -> Switch/1
  x/1 -> Product/2, Add1/1
  Product/1 -> VTHC_CompP_K/1, Add/1  "VTHC_CompP_K"
  Add/1 -> VTHC_CompU_K/1
  Add1/1 -> Unit Delay1/1
  Switch/1 -> Add1/2, Product1/2
  Product1/1 -> Ts/1
  Ts/1 -> VTHC_CompI_K/1, Add/2  "VTHC_CompI_K"
  Unit Delay1/1 -> Switch/3
  Compare To Constant/1 -> Logical Operator/2
  VTHC_CompKp_K/1 -> Product/1
  VTHC_CompKi_K/1 -> Product1/1

== system thc/THC/ThermalControl/THCM_Conctrl/CompCtrl/DeltaUReset ==
  DeltaUin : Inport
  CompPID : Inport  Port=2
  TSetpoint : Inport  Port=3
  Constant1 : Constant  Value=0
  Data Type Conversion : DataTypeConversion  OutDataTypeStr=uint32
  Gain : Gain  Gain=1000
  Logical Operator : Logic  AllPortsSameDT=off  OutDataTypeStr=boolean
  Relational Operator : RelationalOperator  Operator===  OutDataTypeStr=boolean  RndMeth=Simplest
  Relational Operator1 : RelationalOperator  Operator===  OutDataTypeStr=boolean  RndMeth=Simplest
  Switch2 : Switch  Criteria=u2 > Threshold
  Unit Delay : UnitDelay  SampleTime=-1  HasFrameUpgradeWarning=on
  Unit Delay1 : UnitDelay  SampleTime=-1  HasFrameUpgradeWarning=on
  DeltaU : Outport
  wires:
  CompPID/1 -> Relational Operator1/2, Unit Delay/1
  Switch2/1 -> DeltaU/1
  DeltaUin/1 -> Switch2/1
  Constant1/1 -> Switch2/3
  Unit Delay/1 -> Relational Operator1/1
  Logical Operator/1 -> Switch2/2
  Gain/1 -> Data Type Conversion/1
  Unit Delay1/1 -> Relational Operator/1
  Relational Operator/1 -> Logical Operator/2
  Relational Operator1/1 -> Logical Operator/1
  TSetpoint/1 -> Gain/1
  Data Type Conversion/1 -> Unit Delay1/1, Relational Operator/2
